simulink model "untitled1"  (R2023b)
settings: Solver=VariableStepAuto  StartTime=0.0  StopTime=10.0  RelTol=1e-3
values from neighbouring files (symbols this model uses):
  m = size(B2, 2)    [YINF.m]    (also in untitled.m)
libraries: sm_lib x8, nesl_utility x8
settings Model: Creator=A  LastModifiedBy=A

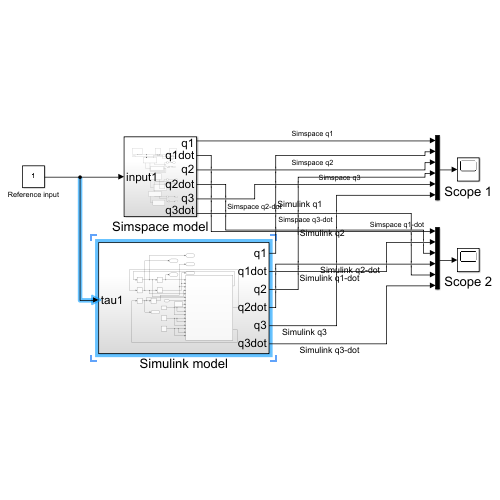
[thumbnail: Simulink's stored preview of the top-level diagram]
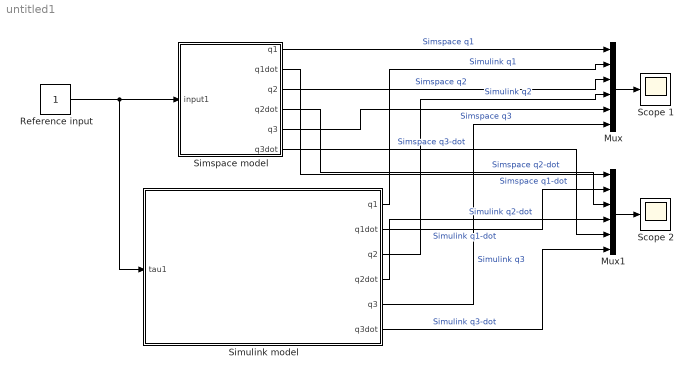
== system untitled1 ==
  Mux : Mux  Inputs=6
  Mux1 : Mux  Inputs=6
  Reference input : Constant
  Scope 1 : Scope
  Scope 2 : Scope
  Simspace model : Subsystem
  Simulink model : Subsystem
  wires:
  Reference input/1 -> Simulink model/1(tau1), Simspace model/1(input1)
  Simulink model/5(q3) -> Mux/6  "Simulink q3"
  Simspace model/3(q2) -> Mux/3  "Simspace q2"
  Simulink model/3(q2) -> Mux/4  "Simulink q2"
  Simspace model/5(q3) -> Mux/5  "Simspace q3"
  Simulink model/2(q1dot) -> Mux1/2  "Simulink q1-dot"
  Simspace model/2(q1dot) -> Mux1/1  "Simspace q1-dot"
  Simulink model/4(q2dot) -> Mux1/4  "Simulink q2-dot"
  Simulink model/6(q3dot) -> Mux1/6  "Simulink q3-dot"
  Simspace model/4(q2dot) -> Mux1/3  "Simspace q2-dot"
  Simspace model/6(q3dot) -> Mux1/5  "Simspace q3-dot"
  Simspace model/1(q1) -> Mux/1  "Simspace q1"
  Simulink model/1(q1) -> Mux/2  "Simulink q1"
  Mux1/1 -> Scope 2/1
  Mux/1 -> Scope 1/1

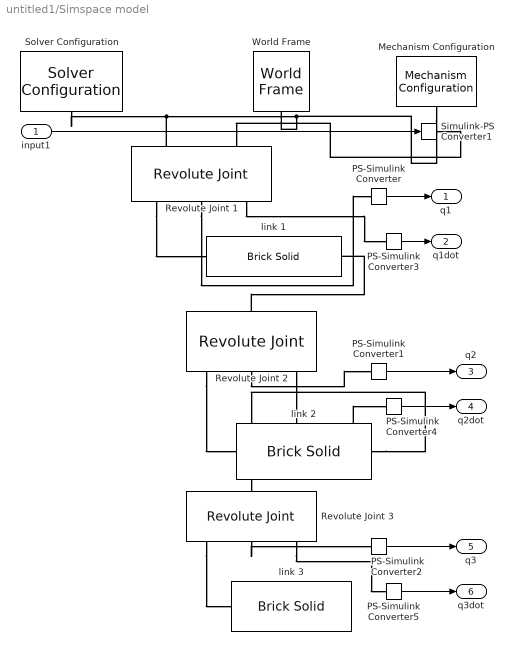
== system untitled1/Simspace model ==
  input1 : Inport
  Mechanism Configuration : sm_lib/Utilities/Mechanism Configuration  UniformGravity=Constant  GravityVector=[0 0 -9.80665]  GravityVectorUnits=m/s^2  LinearizationDelta=0.001  JointModeTransitionNonlinearIterations=2
  PS-Simulink Converter{,1..5} (6 alike) : nesl_utility/PS-Simulink Converter  PhysicalDomain=network_engine_domain  SubClassName=ps_output  LeftPortType=input  RightPortType=output  PseudoPeriodic=off  Frequencies=[]  VectorFormat=inherit  Unit=inherit  AffineConversion=off
  Revolute Joint 1 : sm_lib/Joints/Revolute Joint  JointMode=Normal  SenseConstraintForce=off  SenseConstraintForceX=off  SenseConstraintForceY=off  SenseConstraintForceZ=off  SenseConstraintTorque=off  SenseConstraintTorqueX=off  SenseConstraintTorqueY=off  SenseConstraintTorqueZ=off  SenseTotalForce=off  SenseTotalForceX=off  SenseTotalForceY=off  SenseTotalForceZ=off  SenseTotalTorque=off  SenseTotalTorqueX=off  SenseTotalTorqueY=off  SenseTotalTorqueZ=off  CompositeWrenchDir=FollowerOnBase  CompositeWrenchFrame=BaseFrame  EquilibriumPosition=0  EquilibriumPositionUnits=rad  SpringStiffness=0  SpringStiffnessUnits=N*m/rad  DampingCoefficient=0.05  DampingCoefficientUnits=N*m/(rad/s)  TorqueActuationMode=InputTorque  MotionActuationMode=ComputedMotion  SensePosition=on  SenseVelocity=on  SenseAcceleration=off  SenseTorqueForce=off  SenseLowerLimitTorqueForce=off  SenseUpperLimitTorqueForce=off  LowerLimitSpecify=off  LowerLimitBound=-90  LowerLimitBoundUnits=deg  LowerLimitStiffness=1e4  LowerLimitStiffnessUnits=N*m/deg  LowerLimitDamping=10  LowerLimitDampingUnits=N*m/(deg/s)  LowerLimitTransitionRegionWidth=0.1  LowerLimitTransitionRegionWidthUnits=deg  UpperLimitSpecify=off  UpperLimitBound=90  UpperLimitBoundUnits=deg  UpperLimitStiffness=1e4  UpperLimitStiffnessUnits=N*m/deg  UpperLimitDamping=10  UpperLimitDampingUnits=N*m/(deg/s)  UpperLimitTransitionRegionWidth=0.1  UpperLimitTransitionRegionWidthUnits=deg  PositionTargetSpecify=on  PositionTargetPriority=High  PositionTargetValue=0  PositionTargetValueUnits=deg  VelocityTargetSpecify=on  VelocityTargetPriority=High  VelocityTargetValue=0  VelocityTargetValueUnits=rad/s
  Revolute Joint 2 : sm_lib/Joints/Revolute Joint  JointMode=Normal  SenseConstraintForce=off  SenseConstraintForceX=off  SenseConstraintForceY=off  SenseConstraintForceZ=off  SenseConstraintTorque=off  SenseConstraintTorqueX=off  SenseConstraintTorqueY=off  SenseConstraintTorqueZ=off  SenseTotalForce=off  SenseTotalForceX=off  SenseTotalForceY=off  SenseTotalForceZ=off  SenseTotalTorque=off  SenseTotalTorqueX=off  SenseTotalTorqueY=off  SenseTotalTorqueZ=off  CompositeWrenchDir=FollowerOnBase  CompositeWrenchFrame=BaseFrame  EquilibriumPosition=0  EquilibriumPositionUnits=rad  SpringStiffness=0  SpringStiffnessUnits=N*m/rad  DampingCoefficient=0.05  DampingCoefficientUnits=N*m/(rad/s)  TorqueActuationMode=NoTorque  MotionActuationMode=ComputedMotion  SensePosition=on  SenseVelocity=on  SenseAcceleration=off  SenseTorqueForce=off  SenseLowerLimitTorqueForce=off  SenseUpperLimitTorqueForce=off  LowerLimitSpecify=off  LowerLimitBound=-90  LowerLimitBoundUnits=deg  LowerLimitStiffness=1e4  LowerLimitStiffnessUnits=N*m/deg  LowerLimitDamping=10  LowerLimitDampingUnits=N*m/(deg/s)  LowerLimitTransitionRegionWidth=0.1  LowerLimitTransitionRegionWidthUnits=deg  UpperLimitSpecify=off  UpperLimitBound=90  UpperLimitBoundUnits=deg  UpperLimitStiffness=1e4  UpperLimitStiffnessUnits=N*m/deg  UpperLimitDamping=10  UpperLimitDampingUnits=N*m/(deg/s)  UpperLimitTransitionRegionWidth=0.1  UpperLimitTransitionRegionWidthUnits=deg  PositionTargetSpecify=on  PositionTargetPriority=High  PositionTargetValue=0  PositionTargetValueUnits=deg  VelocityTargetSpecify=off  VelocityTargetPriority=High  VelocityTargetValue=0  VelocityTargetValueUnits=rad/s
  Revolute Joint 3 : sm_lib/Joints/Revolute Joint  JointMode=Normal  SenseConstraintForce=off  SenseConstraintForceX=off  SenseConstraintForceY=off  SenseConstraintForceZ=off  SenseConstraintTorque=off  SenseConstraintTorqueX=off  SenseConstraintTorqueY=off  SenseConstraintTorqueZ=off  SenseTotalForce=off  SenseTotalForceX=off  SenseTotalForceY=off  SenseTotalForceZ=off  SenseTotalTorque=off  SenseTotalTorqueX=off  SenseTotalTorqueY=off  SenseTotalTorqueZ=off  CompositeWrenchDir=FollowerOnBase  CompositeWrenchFrame=BaseFrame  EquilibriumPosition=0  EquilibriumPositionUnits=rad  SpringStiffness=0  SpringStiffnessUnits=N*m/rad  DampingCoefficient=0.05  DampingCoefficientUnits=N*m/(rad/s)  TorqueActuationMode=NoTorque  MotionActuationMode=ComputedMotion  SensePosition=on  SenseVelocity=on  SenseAcceleration=off  SenseTorqueForce=off  SenseLowerLimitTorqueForce=off  SenseUpperLimitTorqueForce=off  LowerLimitSpecify=off  LowerLimitBound=-90  LowerLimitBoundUnits=deg  LowerLimitStiffness=1e4  LowerLimitStiffnessUnits=N*m/deg  LowerLimitDamping=10  LowerLimitDampingUnits=N*m/(deg/s)  LowerLimitTransitionRegionWidth=0.1  LowerLimitTransitionRegionWidthUnits=deg  UpperLimitSpecify=off  UpperLimitBound=90  UpperLimitBoundUnits=deg  UpperLimitStiffness=1e4  UpperLimitStiffnessUnits=N*m/deg  UpperLimitDamping=10  UpperLimitDampingUnits=N*m/(deg/s)  UpperLimitTransitionRegionWidth=0.1  UpperLimitTransitionRegionWidthUnits=deg  PositionTargetSpecify=on  PositionTargetPriority=High  PositionTargetValue=0  PositionTargetValueUnits=deg  VelocityTargetSpecify=off  VelocityTargetPriority=High  VelocityTargetValue=0  VelocityTargetValueUnits=rad/s
  Simulink-PS Converter1 : nesl_utility/Simulink-PS Converter  PhysicalDomain=network_engine_domain  SubClassName=ps_input  LeftPortType=input  RightPortType=output  PseudoPeriodic=off  Frequencies=[]  NoiseDistribution=none  NoiseParameters=[]  Unit=N*m  AffineConversion=off  FilteringAndDerivatives=provide  SimscapeFilterOrder=1  InputFilterTimeConstant=0.001  UdotUserProvided=0
  Solver Configuration : nesl_utility/Solver Configuration  PhysicalDomain=network_engine_domain  SubClassName=solver  LeftPortType=input  RightPortType=generic  Tones=[]  Harmonics=[]  SimulateNoise=off  Profile=off  UseLocalSampling=off  EnableSwitchedLinearOptims=on  FrequencyDomain=off  UseCCode=off  RelTol=0.001  AbsTol=0.001  MinStep=1e-09  ToWorkspace=off  RevertToSquareIcSolve=off  NumHomotopyIterations=100  PhasorMode=off  PhasorModeNumHarmonics=1  ConsistencySolver=NEWTON_XTOL_AFTER_FTOL  IndexReductionMethod=DerivativeReplacement  DoDC=off  ResidualTolerance=1e-09  ConsistencyTolSource=GLOBAL  ConsistencyAbsTol=0.001  ConsistencyRelTol=0.001  ConsistencyTolFactor=0.001  UseLocalSolver=off  LocalSolverChoice=NE_BACKWARD_EULER_ADVANCER  ResolveIndetEquations=on  FunctionEvalNumThread=1  LocalSolverSampleTime=0.001  DoFixedCost=off  MaxNonlinIter=3  MaxModeIter=2  ComputeImpulses=off  ImpulseIterations=2  LinearAlgebra=auto  LinearAlgebraNumThread=0  EquationFormulation=NE_TIME_EF  DelaysMemoryBudget=1024  AutomaticFiltering=on  FilteringTimeConstant=0.001  PartitionStorageMethod=AS_NEEDED  PartitionMemoryBudget=1024  PartitionMethod=ROBUST  MultibodyUseLocalSolver=off  MultibodyLocalSolverChoice=ODE1  MultibodyLocalSolverSampleTime=0.001
  World Frame : sm_lib/Frames and Transforms/World Frame
  link 1 : sm_lib/Body Elements/Brick Solid  GraphicAmbientColor=[0.15 0.15 0.15 1.0]  BasedOnType=Density  BrickDimensions=[0.5 0.02 0.02]  BrickDimensionsUnits=m  CenterOfMass=[0 0 0]  CenterOfMassUnits=m  GraphicDiffuseColor=[0.5 0.5 0.5]  Density=1000  DensityUnits=kg/m^3  DoExposeReferenceFrame=off  GraphicEmissiveColor=[0.0 0.0 0.0 1.0]  ExportEntireGeometry=off  SerializedFrames=<Frames><Frame><Id>Frame1</Id><Value><Name>F1</Name><Origin><Source>GeometricFeature</Source><FeatureName>-x surface</FeatureName></Origin><PrimaryAxis><DefinedDirection>+Z</DefinedDirection><Source>ReferenceFrame</Source><SourceDirection>+Z</SourceDirection><FeatureName></FeatureName></PrimaryAxis><SecondaryAxis><DefinedDirection>+X</DefinedDirection><Source>ReferenceFrame</Source><SourceDirection>+X</SourceDirection><FeatureName></FeatureName></SecondaryAxis></Value></Frame><Frame><Id>Frame2</Id><Value><Name>F2</Name><Origin><Source>GeometricFeature</Source><FeatureName>+x surface</FeatureName></Origin><PrimaryAxis><DefinedDirection>+X</DefinedDirection><Source>ReferenceFrame</Source><SourceDirection>+Z</SourceDirection><FeatureName></FeatureName></PrimaryAxis><SecondaryAxis><DefinedDirection>+Z</DefinedDirection><Source>ReferenceFrame</Source><SourceDirection>+X</SourceDirection><FeatureName></FeatureName></SecondaryAxis></Value></Frame></Frames>  MarkerShape=Sphere  MarkerSize=10  GraphicType=FromGeometry  InertiaType=CalculateFromGeometry  Mass=1  MassUnits=kg  MomentsOfInertia=[1 1 1]  MomentsOfInertiaUnits=kg*m^2  GraphicOpacity=1.0  ProductsOfInertia=[0 0 0]  ProductsOfInertiaUnits=kg*m^2  GraphicShininess=75  GraphicSpecularColor=[0.5 0.5 0.5 1.0]  GraphicVisPropType=SimpleVisualProperties
  link 2 : sm_lib/Body Elements/Brick Solid  GraphicAmbientColor=[0.15 0.15 0.15 1.0]  BasedOnType=Density  BrickDimensions=[0.02 0.02 0.5]  BrickDimensionsUnits=m  CenterOfMass=[0 0 0]  CenterOfMassUnits=m  GraphicDiffuseColor=[1.0 0.8 0.2]  Density=1000  DensityUnits=kg/m^3  DoExposeReferenceFrame=off  GraphicEmissiveColor=[0.0 0.0 0.0 1.0]  ExportEntireGeometry=off  SerializedFrames=<Frames><Frame><Id>Frame1</Id><Value><Name>F1</Name><Origin><Source>GeometricFeature</Source><FeatureName>+z surface</FeatureName></Origin><PrimaryAxis><DefinedDirection>-X</DefinedDirection><Source>ReferenceFrame</Source><SourceDirection>+Z</SourceDirection><FeatureName></FeatureName></PrimaryAxis><SecondaryAxis><DefinedDirection>+Z</DefinedDirection><Source>ReferenceFrame</Source><SourceDirection>+X</SourceDirection><FeatureName></FeatureName></SecondaryAxis></Value></Frame><Frame><Id>Frame2</Id><Value><Name>F2</Name><Origin><Source>GeometricFeature</Source><FeatureName>-z surface</FeatureName></Origin><PrimaryAxis><DefinedDirection>-X</DefinedDirection><Source>ReferenceFrame</Source><SourceDirection>+Z</SourceDirection><FeatureName></FeatureName></PrimaryAxis><SecondaryAxis><DefinedDirection>+Z</DefinedDirection><Source>ReferenceFrame</Source><SourceDirection>+X</SourceDirection><FeatureName></FeatureName></SecondaryAxis></Value></Frame></Frames>  MarkerShape=Sphere  MarkerSize=10  GraphicType=FromGeometry  InertiaType=CalculateFromGeometry  Mass=1  MassUnits=kg  MomentsOfInertia=[1 1 1]  MomentsOfInertiaUnits=kg*m^2  GraphicOpacity=1.0  ProductsOfInertia=[0 0 0]  ProductsOfInertiaUnits=kg*m^2  GraphicShininess=75  GraphicSpecularColor=[0.5 0.5 0.5 1.0]  GraphicVisPropType=SimpleVisualProperties
  link 3 : sm_lib/Body Elements/Brick Solid  GraphicAmbientColor=[0.15 0.15 0.15 1.0]  BasedOnType=Density  BrickDimensions=[0.02 0.02 0.5]  BrickDimensionsUnits=m  CenterOfMass=[0 0 0]  CenterOfMassUnits=m  GraphicDiffuseColor=[0.5 0.5 0.5]  Density=1000  DensityUnits=kg/m^3  DoExposeReferenceFrame=off  GraphicEmissiveColor=[0.0 0.0 0.0 1.0]  ExportEntireGeometry=off  SerializedFrames=<Frames><Frame><Id>Frame1</Id><Value><Name>F1</Name><Origin><Source>GeometricFeature</Source><FeatureName>+z surface</FeatureName></Origin><PrimaryAxis><DefinedDirection>-X</DefinedDirection><Source>ReferenceFrame</Source><SourceDirection>+Z</SourceDirection><FeatureName></FeatureName></PrimaryAxis><SecondaryAxis><DefinedDirection>+Z</DefinedDirection><Source>ReferenceFrame</Source><SourceDirection>+X</SourceDirection><FeatureName></FeatureName></SecondaryAxis></Value></Frame></Frames>  MarkerShape=Sphere  MarkerSize=10  GraphicType=FromGeometry  InertiaType=CalculateFromGeometry  Mass=1  MassUnits=kg  MomentsOfInertia=[1 1 1]  MomentsOfInertiaUnits=kg*m^2  GraphicOpacity=1.0  ProductsOfInertia=[0 0 0]  ProductsOfInertiaUnits=kg*m^2  GraphicShininess=75  GraphicSpecularColor=[0.5 0.5 0.5 1.0]  GraphicVisPropType=SimpleVisualProperties
  q1 : Outport
  q1dot : Outport  Port=2
  q2 : Outport  Port=3
  q2dot : Outport  Port=4
  q3 : Outport  Port=5
  q3dot : Outport  Port=6
  wires:
  input1/1 -> Simulink-PS Converter1/1
  PS-Simulink Converter/1 -> q1/1
  PS-Simulink Converter1/1 -> q2/1
  PS-Simulink Converter2/1 -> q3/1
  PS-Simulink Converter3/1 -> q1dot/1
  PS-Simulink Converter4/1 -> q2dot/1
  PS-Simulink Converter5/1 -> q3dot/1
  connections:
  Solver Configuration/RConn1 -- Mechanism Configuration/RConn1 -- World Frame/RConn1 -- Revolute Joint 1/LConn1
  Revolute Joint 2/RConn2 -- PS-Simulink Converter1/LConn1
  Simulink-PS Converter1/RConn1 -- Revolute Joint 1/LConn2
  Revolute Joint 2/LConn1 -- link 1/RConn1
  Revolute Joint 2/RConn1 -- link 2/LConn1
  Revolute Joint 1/RConn2 -- PS-Simulink Converter/LConn1
  Revolute Joint 1/RConn1 -- link 1/LConn1
  Revolute Joint 3/RConn2 -- PS-Simulink Converter2/LConn1
  Revolute Joint 3/RConn1 -- link 3/LConn1
  link 2/RConn1 -- Revolute Joint 3/LConn1
  Revolute Joint 1/RConn3 -- PS-Simulink Converter3/LConn1
  Revolute Joint 2/RConn3 -- PS-Simulink Converter4/LConn1
  Revolute Joint 3/RConn3 -- PS-Simulink Converter5/LConn1

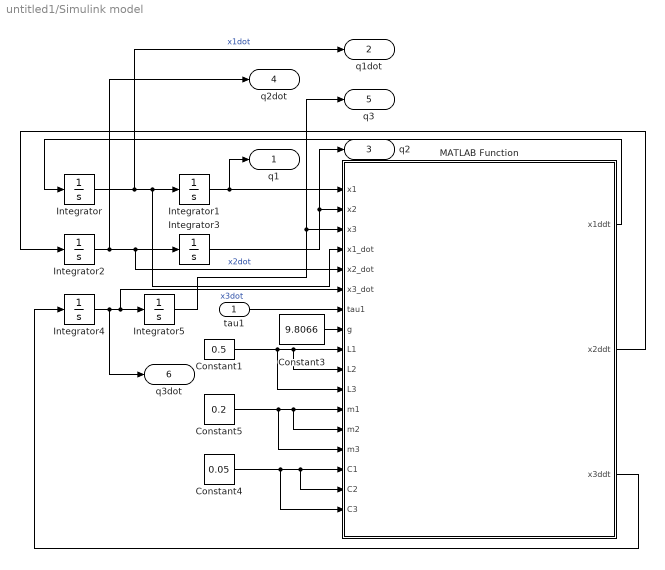
== system untitled1/Simulink model ==
  tau1 : Inport
  Constant1 : Constant  Value=0.5
  Constant3 : Constant  Value=9.8066
  Constant4 : Constant  Value=0.05
  Constant5 : Constant  Value=0.2
  Integrator{,1..5} (6 alike) : Integrator
  MATLAB Function : MATLAB Function  TreatAsAtomicUnit=on
  q1 : Outport
  q1dot : Outport  Port=2
  q2 : Outport  Port=3
  q2dot : Outport  Port=4
  q3 : Outport  Port=5
  q3dot : Outport  Port=6
  wires:
  Integrator4/1 -> Integrator5/1, MATLAB Function/6(x3_dot), q3dot/1  "x3dot"
  Integrator1/1 -> MATLAB Function/1(x1), q1/1
  Constant4/1 -> MATLAB Function/16(C2), MATLAB Function/15(C1), MATLAB Function/17(C3)
  MATLAB Function/2(x2ddt) -> Integrator2/1
  MATLAB Function/1(x1ddt) -> Integrator/1
  Integrator2/1 -> q2dot/1, MATLAB Function/5(x2_dot), Integrator3/1  "x2dot"
  tau1/1 -> MATLAB Function/7(tau1)
  Integrator/1 -> q1dot/1, MATLAB Function/4(x1_dot), Integrator1/1  "x1dot"
  Constant3/1 -> MATLAB Function/8(g)
  Constant5/1 -> MATLAB Function/13(m2), MATLAB Function/12(m1), MATLAB Function/14(m3)
  MATLAB Function/3(x3ddt) -> Integrator4/1
  Integrator3/1 -> q2/1, MATLAB Function/2(x2)
  Integrator5/1 -> q3/1, MATLAB Function/3(x3)
  Constant1/1 -> MATLAB Function/11(L3), MATLAB Function/10(L2), MATLAB Function/9(L1)

== matlab function untitled1/Simulink model/MATLAB Function ==
  data: x1 input; x1ddt output; x2 input; x3 input; x1_dot input; x2_dot input; x3_dot input; tau1 input; g input; x2ddt output; x3ddt output; L1 input; L2 input; L3 input; m1 input; m2 input; m3 input; C1 input; C2 input; C3 input
function [x1ddt,x2ddt,x3ddt] = fcn(x1,x2,x3,x1_dot,x2_dot,x3_dot,tau1,g,L1,L2,L3,m1,m2,m3,C1,C2,C3)

I1=(m1/12)*L1*L1;
I2=(m2/12)*L2*L2;
I3=(m3/12)*L3*L3;

d11=I1 + I2/2 + I3/2 - (I3*cos(2*x2 + 2*x3))/2 + (L1^2*m1)/4 + L1^2*m2 + L1^2*m3 + (L2^2*m2)/8 + (L2^2*m3)/2 + (L3^2*m3)/8 - (I2*cos(2*x2))/2 - (L2^2*m2*cos(2*x2))/8 - (L2^2*m3*cos(2*x2))/2 - (L3^2*m3*cos(2*x2 + 2*x3))/8 + (L2*L3*m3*cos(x3))/2 - (L2*L3*m3*cos(2*x2 + x3))/2;
d12=-(L1*(L3*m3*cos(x2 + x3) + L2*m2*cos(x2) + 2*L2*m3*cos(x2)))/2;
d13=-(L1*L3*m3*cos(x2 + x3))/2;
d21=d12;
d22=I2 + I3 + (L2^2*m2)/4 + L2^2*m3 + (L3^2*m3)/4 + L2*L3*m3*cos(x3);
d23=(m3*L3^2)/4 + (L2*m3*cos(x3)*L3)/2 + I3;
d31=d13;
d32=d23;
d33=(m3*L3^2)/4 + I3;
Dq=[d11,d12,d13;
    d21,d22,d23;
    d31,d32,d33];


c11=I3*x1_dot*x2_dot*sin(2*x2 + 2*x3) + I3*x1_dot*x3_dot*sin(2*x2 + 2*x3) + I2*x1_dot*x2_dot*sin(2*x2) + (L1*L2*m2*x2_dot^2*sin(x2))/2 + L1*L2*m3*x2_dot^2*sin(x2) + (L2^2*m2*x1_dot*x2_dot*sin(2*x2))/4 + L2^2*m3*x1_dot*x2_dot*sin(2*x2) + (L3^2*m3*x1_dot*x2_dot*sin(2*x2 + 2*x3))/4 + (L3^2*m3*x1_dot*x3_dot*sin(2*x2 + 2*x3))/4 + (L1*L3*m3*x2_dot^2*sin(x2 + x3))/2 + (L1*L3*m3*x3_dot^2*sin(x2 + x3))/2 + L1*L3*m3*x2_dot*x3_dot*sin(x2 + x3) - (L2*L3*m3*x1_dot*x3_dot*sin(x3))/2 + L2*L3*m3*x1_dot*x2_dot*sin(2*x2 + x3) + (L2*L3*m3*x1_dot*x3_dot*sin(2*x2 + x3))/2;
c21= -(I3*x1_dot^2*sin(2*x2 + 2*x3))/2 - (I2*x1_dot^2*sin(2*x2))/2 - (L2^2*m2*x1_dot^2*sin(2*x2))/8 - (L2^2*m3*x1_dot^2*sin(2*x2))/2 - (L3^2*m3*x1_dot^2*sin(2*x2 + 2*x3))/8 - (L2*L3*m3*x3_dot^2*sin(x3))/2 - (L2*L3*m3*x1_dot^2*sin(2*x2 + x3))/2 - L2*L3*m3*x2_dot*x3_dot*sin(x3);
c31= ((L2*L3*m3*sin(x3))/4 - (L3^2*m3*sin(2*x2 + 2*x3))/8 - (I3*sin(2*x2 + 2*x3))/2 - (L2*L3*m3*sin(2*x2 + x3))/4)*x1_dot^2 + (L2*L3*m3*sin(x3)*x2_dot^2)/2;
cq=[c11;
    c21;
    c31];

g11=0;
g21=- g*m3*((L3*sin(x2 + x3))/2 + L2*sin(x2)) - (L2*g*m2*sin(x2))/2;
g31=-(L3*g*m3*sin(x2 + x3))/2;
Gq=[g11;
    g21;
    g31];

W11=C1*x1_dot;
W21=C2*x2_dot;
W31=C3*x3_dot;
Fi=[W11;
    W21;
    W31];

tau=[tau1;
    0;
    0];

ddx = Dq \ (tau - cq - Gq - Fi);
x1ddt=ddx(1,:);
x2ddt=ddx(2,:);
x3ddt=ddx(3,:);
